simulink model "BlackBoxModel"  (R2024b)
settings: Solver=VariableStepAuto  StartTime=0.0  StopTime=10.0  RelTol=1e-3
InitFcn:
  | Init
StopFcn:
  | Plotting
values from neighbouring files (symbols this model uses):
  degs2rpm = 60/360    (= 0.166666666667)    [Init.m]    (also in ModelParams.m; load_params_inertial_case.m)
  delta_est = 1/sqrt(2)    [Init.m]    (also in code.m; main.m)
  Kd = Kp * Td    [Init.m]    (also in code.m; main.m)
  Ki = Kp / Ti    [Init.m]    (also in code.m; main.m)
  Kp = deltak * cos(deltaphi)    [Init.m]    (also in code.m = deltak*cos(deltaphi); main.m = deltak*cos(deltaphi))
  rpm2degs = 360/60    (= 6)    [Init.m]    (also in ModelParams.m; load_params_inertial_case.m)
  rpm2rads = 2*pi/60    (= 0.10471975512)    [Init.m]    (also in ModelParams.m; load_params_inertial_case.m)
  tl = 1/(3*wgc)    [Init.m]    (also in code.m = 1/cut_off; main.m = 1/cut_off)
  wc = 2*pi*20    (= 125.663706144)    [Init.m]    (also in code.m; main.m)
undefined symbols (not defined in the file or in its folder): gbox, mld, mot, sens
settings Model: Creator=Banaan  LastModifiedBy=Banaan
settings DebuggingCC: AlgebraicLoopMsg=none

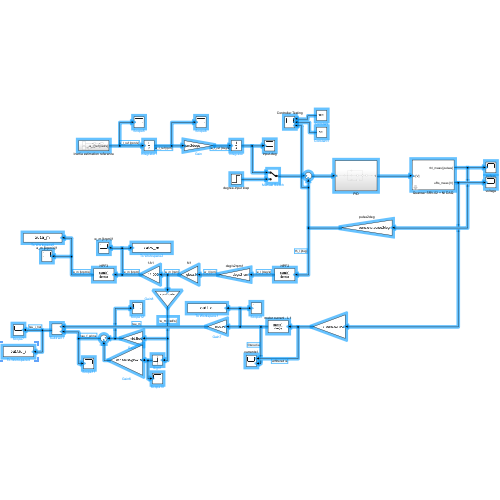
[thumbnail: Simulink's stored preview of the top-level diagram]
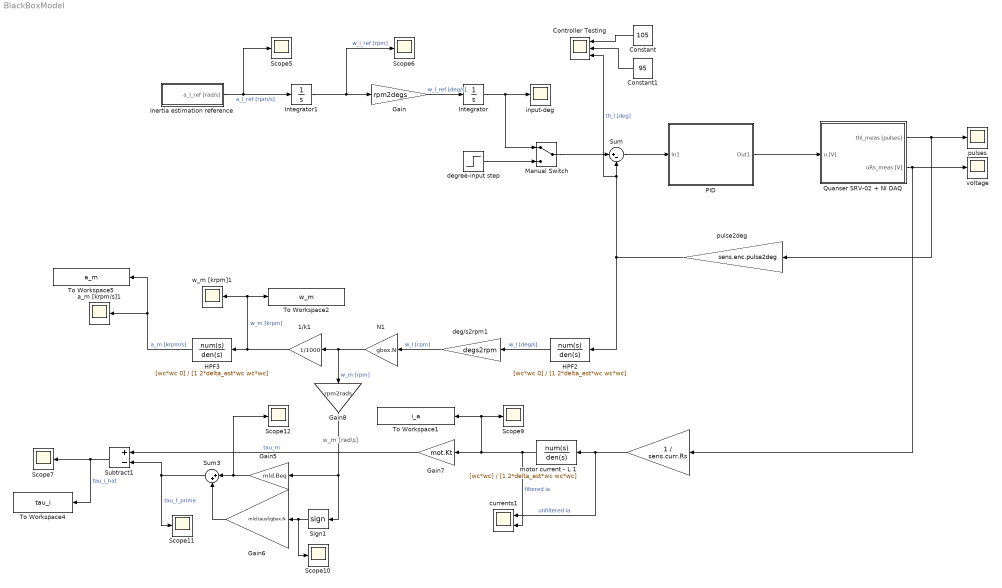
== system BlackBoxModel ==
  note: w_m [rad\s]
  " " : Gain  Gain=1 / sens.curr.Rs
  1/k1 : Gain  Gain=1/1000
  Constant : Constant  Value=105
  Constant1 : Constant  Value=95
  Controller Testing : Scope  NumInputPorts=3
  Gain : Gain  Gain=rpm2degs
  Gain5 : Gain  Gain=mld.Beq
  Gain6 : Gain  Gain=mld.tausf/gbox.N
  Gain7 : Gain  Gain=mot.Kt
  Gain8 : Gain  Gain=rpm2rads
  HPF2 : TransferFcn  Numerator=[wc*wc 0]  Denominator=[1 2*delta_est*wc wc*wc]
  HPF3 : TransferFcn  Numerator=[wc*wc 0]  Denominator=[1 2*delta_est*wc wc*wc]
  Inertia estimation reference : Subsystem
  Integrator : Integrator
  Integrator1 : Integrator
  Manual Switch : ManualSwitch
  N1 : Gain  Gain=gbox.N
  PID : Subsystem
  Quanser SRV-02 + NI DAQ : Subsystem  mask(Quanser SRV-02 (with inertial load) + NI DAQ){Ts=0.001, fricType=Coulomb + viscous}
      mask prompts: Ts "NI DAQ Sample Time:"; fricType "Friction model"
      mask help: Quanser SRV-02 (with inertial load) + NI DAQ model.
      mask init:
      | %%  Sensors data
      | 
      | %   shunt resistor
      | sens.curr.Rs = 0.5;                         %   resistance [Ohm]   
      | sens.curr.uRs_std = 0.01;                   %   voltage noise standard dev [V]                           
      | sens.curr.uRs_var = sens.curr.uRs_std^2;	%   voltage noise variance [V^2]
      | 
      | %   Hewlett-Packard HEDS-5540#A06 optical encoder
      | sens.enc.ppr = 500*4;                       %   pulses per rotation
      | sens.enc.pulse2deg = 360/sens.enc.ppr;      %   [pulses] -> [deg]
      | sens.enc.pulse2rad = 2*pi/sens.enc.ppr;     %   [pulses] -> [rad]
      | sens.enc.deg2pulse = sens.enc.ppr/360;      %   [deg] -> [pulses]
      | sens.enc.rad2pulse = sens.enc.ppr/2/pi;     %   [rad] -> [pulses]
      | 
      | 
      | %%  Data acquisition board (daq) data
      | 
      | %   NI PCI-6221 DAC data
      | daq.dac.bits = 16;                                  %   resolution (bits)
      | daq.dac.fs   = 10;                                  %   full scale 
      | daq.dac.q    = 2*daq.dac.fs/(2^daq.dac.bits-1);     %	quantization
      | 
      | %   NI PCI-6221 ADC data
      | daq.adc.bits = 16;                                  %   resolution (bits)
      | daq.adc.fs   = 10;                                  %   full scale (as set in SLDRT Analog Input block)
      | daq.adc.q    = 2*daq.adc.fs/(2^daq.adc.bits-1);     %   quantization
      mask Help:
      | Riccardo Antonello (antonello@dei.unipd.it)
      | 
      | April 24, 2020
      | 
      | Dept. of Information Engineering, University of Padova
      mask TypeOptions fricType: Coulomb + viscous | Karnopp
  Scope{5..7,9..12} (7 alike) : Scope
  Sign1 : Signum  ZeroCross=off
  Subtract1 : Sum  Inputs=+-
  Sum : Sum  Inputs=|+-
  Sum3 : Sum  Inputs=|++
  To Workspace1 : ToWorkspace  VariableName=i_a  SaveFormat=Structure With Time  SampleTime=-1
  To Workspace2 : ToWorkspace  VariableName=w_m  SaveFormat=Structure With Time  SampleTime=-1
  To Workspace4 : ToWorkspace  VariableName=tau_i  SaveFormat=Structure With Time  SampleTime=-1
  To Workspace5 : ToWorkspace  VariableName=a_m  SaveFormat=Structure With Time  SampleTime=-1
  a_m [krpm/s]1 : Scope
  currents1 : Scope  NumInputPorts=2
  deg/s2rpm1 : Gain  Gain=degs2rpm
  degree-input step : Step  Time=0  After=100  SampleTime=0
  input-deg : Scope
  motor current - L 1 : TransferFcn  Numerator=[wc*wc]  Denominator=[1 2*delta_est*wc wc*wc]
  pulse2deg : Gain  Gain=sens.enc.pulse2deg
  pulses : Scope
  voltage : Scope
  w_m [krpm]1 : Scope
  wires:
  Sum/1 -> PID/1(In1)
  Manual Switch/1 -> Sum/1
  Integrator/1 -> Manual Switch/1, input-deg/1
  degree-input step/1 -> Manual Switch/2
  Quanser SRV-02 + NI DAQ/1(thl_meas [pulses]) -> pulses/1, pulse2deg/1
  PID/1(Out1) -> Quanser SRV-02 + NI DAQ/1(u [V])
  Constant/1 -> Controller Testing/1
  Constant1/1 -> Controller Testing/2
  Integrator1/1 -> Scope6/1, Gain/1  "w_l_ref [rpm]"
  Gain/1 -> Integrator/1  "w_l_ref [deg/s]"
  Inertia estimation reference/1(a_l_ref [rad/s]) -> Scope5/1, Integrator1/1  "a_l_ref [rpm/s]"
  HPF3/1 -> a_m [krpm/s]1/1, To Workspace5/1  "a_m [krpm/s]"
  N1/1 -> Gain8/1, 1/k1/1  "w_m [rpm]"
  Gain5/1 -> Sum3/1, Scope12/1
  Gain8/1 -> Sign1/1, Gain5/1
  pulse2deg/1 -> HPF2/1, Controller Testing/3, Sum/2  "th_l [deg]"
  Sum3/1 -> Subtract1/2, Scope11/1  "tau_f_prime"
  Gain6/1 -> Sum3/2
  1/k1/1 -> HPF3/1, To Workspace2/1, w_m [krpm]1/1  "w_m [krpm]"
  HPF2/1 -> deg/s2rpm1/1  "w_l [deg/s]"
  motor current - L 1/1 -> To Workspace1/1, Scope9/1, Gain7/1, currents1/2  "filtered ia"
  " "/1 -> currents1/1, motor current - L 1/1  "unfiltered ia"
  Sign1/1 -> Scope10/1, Gain6/1
  Subtract1/1 -> To Workspace4/1, Scope7/1  "tau_i_hat"
  Quanser SRV-02 + NI DAQ/2(uRs_meas [V]) -> voltage/1, " "/1
  Gain7/1 -> Subtract1/1  "tau_m"
  deg/s2rpm1/1 -> N1/1  "w_l [rpm]"

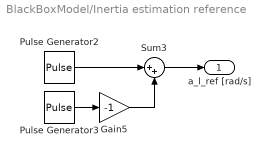
== system BlackBoxModel/Inertia estimation reference ==
  Gain5 : Gain  Gain=-1
  Pulse Generator2 : DiscretePulseGenerator  PulseType=Time based  Amplitude=450  PulseWidth=50
  Pulse Generator3 : DiscretePulseGenerator  PulseType=Time based  Amplitude=450  PulseWidth=50  PhaseDelay=1
  Sum3 : Sum  Inputs=|++
  a_l_ref [rad/s] : Outport
  wires:
  Pulse Generator3/1 -> Gain5/1
  Pulse Generator2/1 -> Sum3/1
  Gain5/1 -> Sum3/2
  Sum3/1 -> a_l_ref [rad/s]/1

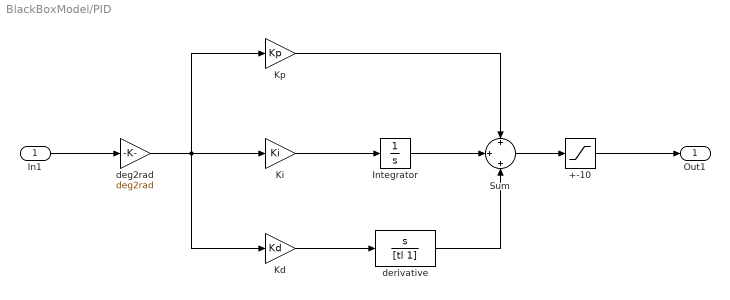
== system BlackBoxModel/PID ==
  In1 : Inport
  +-10 : Saturate  UpperLimit=10  LowerLimit=-10
  Integrator : Integrator
  Kd : Gain  Gain=Kd
  Ki : Gain  Gain=Ki
  Kp : Gain  Gain=Kp
  Sum : Sum  Inputs=+|+|+
  deg2rad : Gain  Gain=deg2rad
  derivative : TransferFcn  Numerator=[1 0]  Denominator=[tl 1]
  Out1 : Outport
  wires:
  In1/1 -> deg2rad/1
  deg2rad/1 -> Kd/1, Kp/1, Ki/1
  Ki/1 -> Integrator/1
  Kp/1 -> Sum/1
  Integrator/1 -> Sum/2
  Kd/1 -> derivative/1
  derivative/1 -> Sum/3
  Sum/1 -> +-10/1
  +-10/1 -> Out1/1

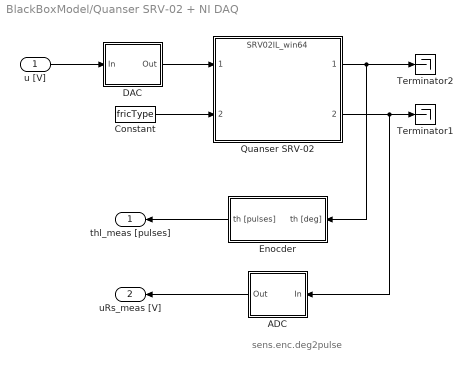
== system BlackBoxModel/Quanser SRV-02 + NI DAQ ==
  note: sens.enc.deg2pulse
  u [V] : Inport
  ADC : Subsystem
  Constant : Constant  Value=fricType
  DAC : Subsystem
  Enocder : Subsystem
  Quanser SRV-02 : ModelReference  ModelNameDialog=SRV02IL_win64.slxp  ModelReferenceVersion=1.44  CopyOfModelProtected=on
  Terminator1 : Terminator
  Terminator2 : Terminator
  thl_meas [pulses] : Outport
  uRs_meas [V] : Outport  Port=2
  wires:
  Enocder/1(th [pulses]) -> thl_meas [pulses]/1
  ADC/1(Out) -> uRs_meas [V]/1
  DAC/1(Out) -> Quanser SRV-02/1
  Quanser SRV-02/2 -> ADC/1(In), Terminator1/1
  u [V]/1 -> DAC/1(In)
  Quanser SRV-02/1 -> Enocder/1(th [deg]), Terminator2/1
  Constant/1 -> Quanser SRV-02/2

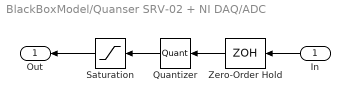
== system BlackBoxModel/Quanser SRV-02 + NI DAQ/ADC ==
  In : Inport
  Quantizer : Quantizer  QuantizationInterval=daq.adc.q
  Saturation : Saturate  UpperLimit=daq.adc.fs  LowerLimit=-daq.adc.fs
  Zero-Order Hold : ZeroOrderHold  SampleTime=Ts
  Out : Outport
  wires:
  Saturation/1 -> Out/1
  In/1 -> Zero-Order Hold/1
  Quantizer/1 -> Saturation/1
  Zero-Order Hold/1 -> Quantizer/1

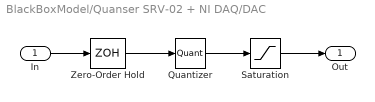
== system BlackBoxModel/Quanser SRV-02 + NI DAQ/DAC ==
  In : Inport
  Quantizer : Quantizer  QuantizationInterval=daq.dac.q
  Saturation : Saturate  UpperLimit=daq.dac.fs  LowerLimit=-daq.dac.fs
  Zero-Order Hold : ZeroOrderHold  SampleTime=Ts
  Out : Outport
  wires:
  Quantizer/1 -> Saturation/1
  In/1 -> Zero-Order Hold/1
  Zero-Order Hold/1 -> Quantizer/1
  Saturation/1 -> Out/1

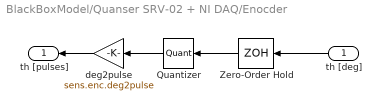
== system BlackBoxModel/Quanser SRV-02 + NI DAQ/Enocder ==
  th [deg] : Inport
  Quantizer : Quantizer  QuantizationInterval=sens.enc.pulse2deg
  Zero-Order Hold : ZeroOrderHold  SampleTime=Ts
  deg2pulse : Gain  Gain=sens.enc.deg2pulse
  th [pulses] : Outport
  wires:
  Quantizer/1 -> deg2pulse/1
  th [deg]/1 -> Zero-Order Hold/1
  Zero-Order Hold/1 -> Quantizer/1
  deg2pulse/1 -> th [pulses]/1
